simulink model "Figure7"  (R2021b)
settings: Solver=VariableStepAuto  StartTime=0.0  StopTime=10.0  RelTol=1e-3
undefined symbols (not defined in the file or in its folder): get, gray, res
libraries: myLib_CustomBoolean x45, dspobslib x1
settings Model: Creator=matt  LastModifiedBy=matt

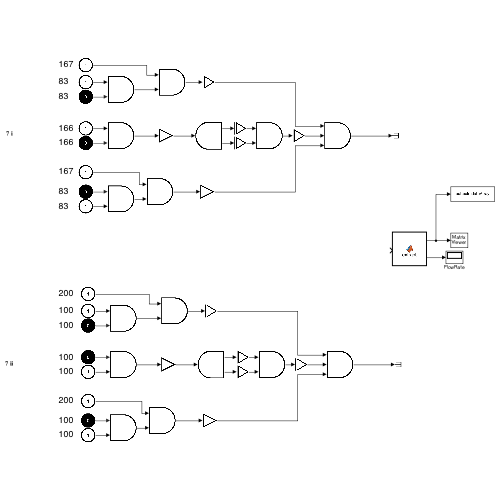
[thumbnail: Simulink's stored preview of the top-level diagram]
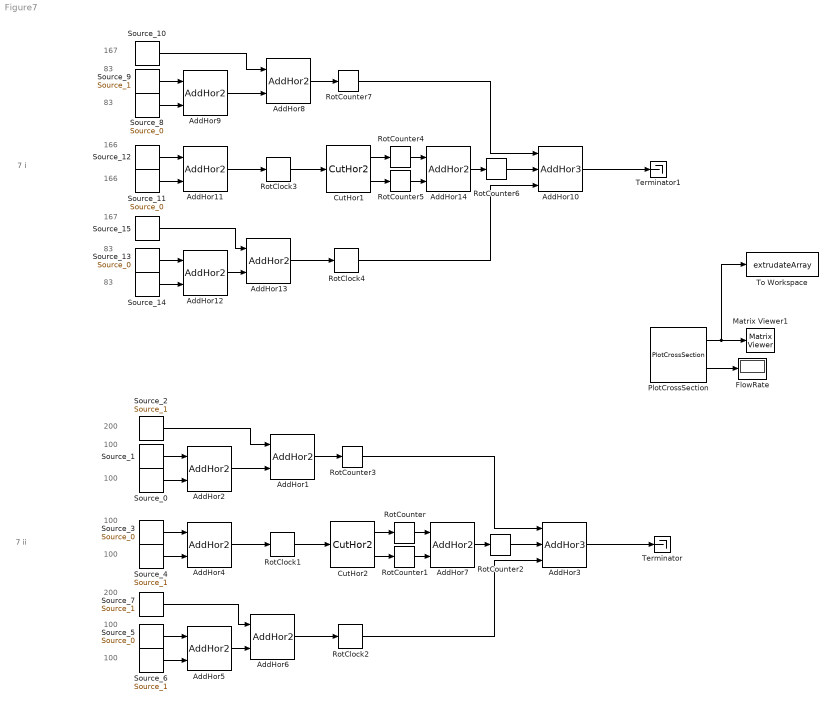
== system Figure7 ==
  note: 7 i
  note: 83
  note: 166
  note: 167
  note: 83
  note: 83
  note: 166
  note: 83
  note: 167
  note: 100
  note: 200
  note: 100
  note: 100
  note: 200
  note: 100
  note: 100
  note: 100
  note: 7 ii
  AddHor{1..2,4..9,11..14} (12 alike) : myLib_CustomBoolean/AddHor2  SystemSampleTime=-1  VariantActivationTime=update diagram  Latency=0  AutoFrameSizeCalculation=off
      settings: SourceProductName=Boolean_Custom_Library
  AddHor10 : myLib_CustomBoolean/AddHor3  SystemSampleTime=-1  VariantActivationTime=update diagram  Latency=0  AutoFrameSizeCalculation=off
      settings: SourceProductName=Boolean_Custom_Library
  AddHor3 : myLib_CustomBoolean/AddHor3  SystemSampleTime=-1  VariantActivationTime=update diagram  Latency=0  AutoFrameSizeCalculation=off
      settings: SourceProductName=Boolean_Custom_Library
  CutHor1 : myLib_CustomBoolean/CutHor2  SystemSampleTime=-1  VariantActivationTime=update diagram  Latency=0  AutoFrameSizeCalculation=off
      settings: SourceProductName=Boolean_Custom_Library
  CutHor2 : myLib_CustomBoolean/CutHor2  SystemSampleTime=-1  VariantActivationTime=update diagram  Latency=0  AutoFrameSizeCalculation=off
      settings: SourceProductName=Boolean_Custom_Library
  FlowRate : Display
  Matrix Viewer1 : dspobslib/Matrix Viewer  ImageParams=off  CMapStr=gray(3)  AxisColorbar=off  AxisParams=off  AxisOrigin=Upper left corner  AxisTickMode=User-defined  XTickRange=[0 1]  YTickRange=[0 1]  XLabel=X-axis  YLabel=Y-axis  ZLabel=Z-axis  FigPos=get(0,'defaultfigureposition')  AxisZoom=off
      settings: SourceProductBaseCode=DS  YMin=0  YMax=1
  PlotCrossSection : myLib_CustomBoolean/PlotCrossSection  SystemSampleTime=-1  VariantActivationTime=update diagram  Latency=0  AutoFrameSizeCalculation=off
      settings: SourceProductName=Boolean_Custom_Library
  RotClock{1..4} (4 alike) : myLib_CustomBoolean/RotClock  SystemSampleTime=-1  VariantActivationTime=update diagram  Latency=0  AutoFrameSizeCalculation=off
      settings: SourceProductName=Boolean_Custom_Library
  RotCounter{,1..7} (8 alike) : myLib_CustomBoolean/RotCounter  SystemSampleTime=-1  VariantActivationTime=update diagram  Latency=0  AutoFrameSizeCalculation=off
      settings: SourceProductName=Boolean_Custom_Library
  Source_0 : myLib_CustomBoolean/Source_0  Value=cat(3, 0.*ones(res,res), 100.*ones(res,res))  VectorParams1D=off  OutMin=[]  OutMax=[]  OutDataTypeStr=Inherit: Inherit from 'Constant value'  SampleTime=inf  FramePeriod=inf
      settings: SourceProductName=Boolean_Custom_Library
  Source_1 : myLib_CustomBoolean/Source_1  Value=cat(3, 1.*ones(res,res), 100*ones(res,res))  VectorParams1D=off  OutMin=[]  OutMax=[]  OutDataTypeStr=Inherit: Inherit from 'Constant value'  SampleTime=inf  FramePeriod=inf
      settings: SourceProductName=Boolean_Custom_Library
  Source_10 : myLib_CustomBoolean/Source_1  Value=cat(3, 1.*ones(res,res), 167.*ones(res,res))  VectorParams1D=off  OutMin=[]  OutMax=[]  OutDataTypeStr=Inherit: Inherit from 'Constant value'  SampleTime=inf  FramePeriod=inf
      settings: SourceProductName=Boolean_Custom_Library
  Source_11 : myLib_CustomBoolean/Source_0  Value=cat(3, 0.*ones(res,res), 166.*ones(res,res))  VectorParams1D=off  OutMin=[]  OutMax=[]  OutDataTypeStr=Inherit: Inherit from 'Constant value'  SampleTime=inf  FramePeriod=inf
      settings: SourceProductName=Boolean_Custom_Library
  Source_12 : myLib_CustomBoolean/Source_1  Value=cat(3, 1.*ones(res,res), 166*ones(res,res))  VectorParams1D=off  OutMin=[]  OutMax=[]  OutDataTypeStr=Inherit: Inherit from 'Constant value'  SampleTime=inf  FramePeriod=inf
      settings: SourceProductName=Boolean_Custom_Library
  Source_13 : myLib_CustomBoolean/Source_0  Value=cat(3, 0.*ones(res,res), 83.*ones(res,res))  VectorParams1D=off  OutMin=[]  OutMax=[]  OutDataTypeStr=Inherit: Inherit from 'Constant value'  SampleTime=inf  FramePeriod=inf
      settings: SourceProductName=Boolean_Custom_Library
  Source_14 : myLib_CustomBoolean/Source_1  Value=cat(3, 1.*ones(res,res), 83*ones(res,res))  VectorParams1D=off  OutMin=[]  OutMax=[]  OutDataTypeStr=Inherit: Inherit from 'Constant value'  SampleTime=inf  FramePeriod=inf
      settings: SourceProductName=Boolean_Custom_Library
  Source_15 : myLib_CustomBoolean/Source_1  Value=cat(3, 1.*ones(res,res), 167*ones(res,res))  VectorParams1D=off  OutMin=[]  OutMax=[]  OutDataTypeStr=Inherit: Inherit from 'Constant value'  SampleTime=inf  FramePeriod=inf
      settings: SourceProductName=Boolean_Custom_Library
  Source_2 : myLib_CustomBoolean/Source_1  Value=cat(3, 1.*ones(res,res), 200*ones(res,res))  VectorParams1D=off  OutMin=[]  OutMax=[]  OutDataTypeStr=Inherit: Inherit from 'Constant value'  SampleTime=inf  FramePeriod=inf
      settings: SourceProductName=Boolean_Custom_Library
  Source_3 : myLib_CustomBoolean/Source_0  Value=cat(3, 0.*ones(res,res), 100.*ones(res,res))  VectorParams1D=off  OutMin=[]  OutMax=[]  OutDataTypeStr=Inherit: Inherit from 'Constant value'  SampleTime=inf  FramePeriod=inf
      settings: SourceProductName=Boolean_Custom_Library
  Source_4 : myLib_CustomBoolean/Source_1  Value=cat(3, 1.*ones(res,res), 100*ones(res,res))  VectorParams1D=off  OutMin=[]  OutMax=[]  OutDataTypeStr=Inherit: Inherit from 'Constant value'  SampleTime=inf  FramePeriod=inf
      settings: SourceProductName=Boolean_Custom_Library
  Source_5 : myLib_CustomBoolean/Source_0  Value=cat(3, 0.*ones(res,res), 100.*ones(res,res))  VectorParams1D=off  OutMin=[]  OutMax=[]  OutDataTypeStr=Inherit: Inherit from 'Constant value'  SampleTime=inf  FramePeriod=inf
      settings: SourceProductName=Boolean_Custom_Library
  Source_6 : myLib_CustomBoolean/Source_1  Value=cat(3, 1.*ones(res,res), 100*ones(res,res))  VectorParams1D=off  OutMin=[]  OutMax=[]  OutDataTypeStr=Inherit: Inherit from 'Constant value'  SampleTime=inf  FramePeriod=inf
      settings: SourceProductName=Boolean_Custom_Library
  Source_7 : myLib_CustomBoolean/Source_1  Value=cat(3, 1.*ones(res,res), 200*ones(res,res))  VectorParams1D=off  OutMin=[]  OutMax=[]  OutDataTypeStr=Inherit: Inherit from 'Constant value'  SampleTime=inf  FramePeriod=inf
      settings: SourceProductName=Boolean_Custom_Library
  Source_8 : myLib_CustomBoolean/Source_0  Value=cat(3, 0.*ones(res,res), 83.*ones(res,res))  VectorParams1D=off  OutMin=[]  OutMax=[]  OutDataTypeStr=Inherit: Inherit from 'Constant value'  SampleTime=inf  FramePeriod=inf
      settings: SourceProductName=Boolean_Custom_Library
  Source_9 : myLib_CustomBoolean/Source_1  Value=cat(3, 1.*ones(res,res), 83*ones(res,res))  VectorParams1D=off  OutMin=[]  OutMax=[]  OutDataTypeStr=Inherit: Inherit from 'Constant value'  SampleTime=inf  FramePeriod=inf
      settings: SourceProductName=Boolean_Custom_Library
  Terminator : Terminator
  Terminator1 : Terminator
  To Workspace : ToWorkspace  VariableName=extrudateArray  SampleTime=51
  wires:
  Source_12/1 -> AddHor11/1
  Source_14/1 -> AddHor12/2
  AddHor13/1 -> RotClock4/1
  RotCounter6/1 -> AddHor10/2
  Source_9/1 -> AddHor9/1
  AddHor14/1 -> RotCounter6/1
  RotCounter5/1 -> AddHor14/2
  AddHor8/1 -> RotCounter7/1
  AddHor9/1 -> AddHor8/2
  AddHor12/1 -> AddHor13/2
  Source_11/1 -> AddHor11/2
  Source_13/1 -> AddHor12/1
  Source_15/1 -> AddHor13/1
  RotCounter4/1 -> AddHor14/1
  CutHor1/2 -> RotCounter5/1
  Source_10/1 -> AddHor8/1
  PlotCrossSection/1 -> Matrix Viewer1/1, To Workspace/1
  AddHor11/1 -> RotClock3/1
  RotCounter7/1 -> AddHor10/1
  CutHor1/1 -> RotCounter4/1
  AddHor10/1 -> Terminator1/1
  RotClock3/1 -> CutHor1/1
  RotClock4/1 -> AddHor10/3
  Source_8/1 -> AddHor9/2
  PlotCrossSection/2 -> FlowRate/1
  RotCounter/1 -> AddHor7/1
  CutHor2/2 -> RotCounter1/1
  AddHor2/1 -> AddHor1/2
  Source_0/1 -> AddHor2/2
  AddHor1/1 -> RotCounter3/1
  Source_5/1 -> AddHor5/1
  Source_7/1 -> AddHor6/1
  RotCounter2/1 -> AddHor3/2
  RotCounter1/1 -> AddHor7/2
  AddHor3/1 -> Terminator/1
  AddHor5/1 -> AddHor6/2
  AddHor7/1 -> RotCounter2/1
  Source_1/1 -> AddHor2/1
  Source_6/1 -> AddHor5/2
  AddHor6/1 -> RotClock2/1
  RotCounter3/1 -> AddHor3/1
  Source_3/1 -> AddHor4/1
  RotClock1/1 -> CutHor2/1
  Source_4/1 -> AddHor4/2
  AddHor4/1 -> RotClock1/1
  CutHor2/1 -> RotCounter/1
  Source_2/1 -> AddHor1/1
  RotClock2/1 -> AddHor3/3
